simulink model "HomeAssignmentSimulinkConstants"  (R2022b)
settings: Solver=VariableStepAuto  StartTime=0.0  StopTime=6  RelTol=1e-3
settings Model: Creator=probo  LastModifiedBy=Nicher
settings DebuggingCC: UnconnectedInputMsg=warning  UnconnectedOutputMsg=warning  UnconnectedLineMsg=warning
settings ModelReferenceCC: EnableRefExpFcnMdlSchedulingChecks=on
settings RTWCC: DLArmComputeVersion=19.05

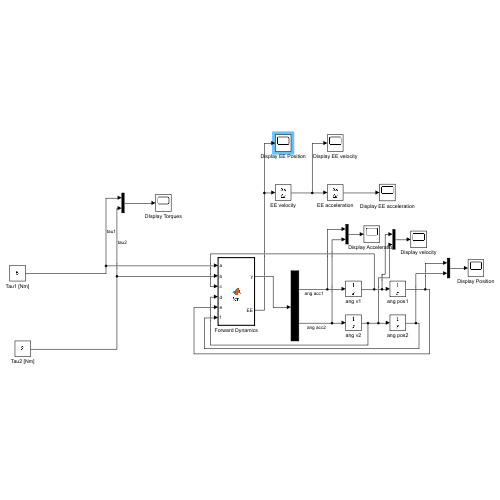
[thumbnail: Simulink's stored preview of the top-level diagram]
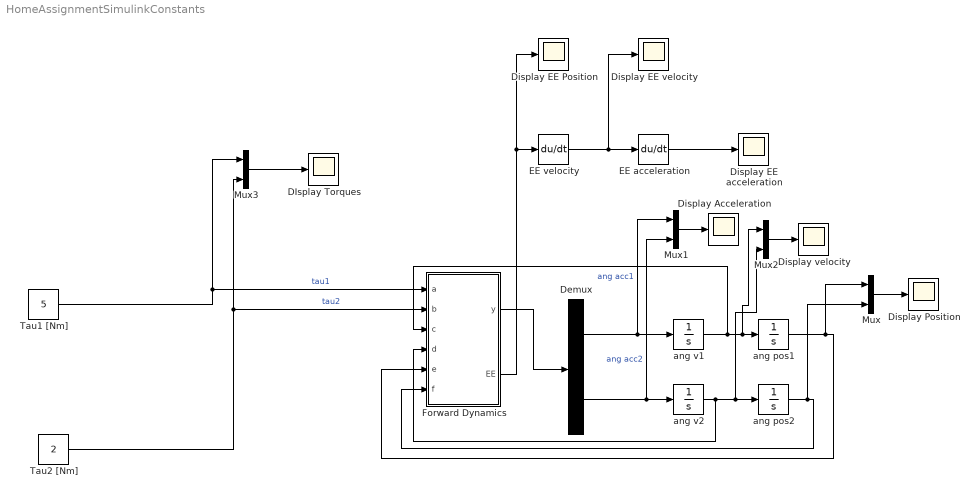
== system HomeAssignmentSimulinkConstants ==
  DIsplay Torques : Scope
  Demux : Demux  Outputs=2
  Display Acceleration : Scope
  Display EE Position : Scope
  Display EE acceleration : Scope
  Display EE velocity : Scope
  Display Position : Scope
  Display velocity : Scope
  EE acceleration : Derivative
  EE velocity : Derivative
  Forward Dynamics : MATLAB Function  TreatAsAtomicUnit=on
  Mux{,1..3} (4 alike) : Mux  Inputs=2
  Tau1 [Nm] : Constant  Value=5
  Tau2 [Nm] : Constant  Value=2
  ang pos1 : Integrator
  ang pos2 : Integrator
  ang v1 : Integrator
  ang v2 : Integrator
  wires:
  Forward Dynamics/1(y) -> Demux/1
  Demux/1 -> Mux1/1, ang v1/1  "ang acc1"
  Demux/2 -> Mux1/2, ang v2/1  "ang acc2"
  ang v1/1 -> Forward Dynamics/3(c), Mux2/1, ang pos1/1
  ang v2/1 -> Forward Dynamics/4(d), ang pos2/1, Mux2/2
  ang pos2/1 -> Mux/2, Forward Dynamics/6(f)
  ang pos1/1 -> Mux/1, Forward Dynamics/5(e)
  Mux1/1 -> Display Acceleration/1
  Mux2/1 -> Display velocity/1
  Tau2 [Nm]/1 -> Forward Dynamics/2(b), Mux3/2  "tau2"
  Tau1 [Nm]/1 -> Forward Dynamics/1(a), Mux3/1  "tau1"
  Mux3/1 -> DIsplay Torques/1
  Mux/1 -> Display Position/1
  Forward Dynamics/2(EE) -> Display EE Position/1, EE velocity/1
  EE velocity/1 -> Display EE velocity/1, EE acceleration/1
  EE acceleration/1 -> Display EE acceleration/1

== matlab function HomeAssignmentSimulinkConstants/Forward Dynamics ==
  data: a input; y output; b input; c input; d input; e input; f input; EE output
function [y, EE]= fcn(a, b, c, d, e, f)

% Torques

tau1 = a;
tau2 = b;

% Joint Velocity & Position

dtheta1 = c;
theta1 = e;

dtheta2 = d;
theta2 = f;

%Variables for link 1
l1 = 0.5;
m1 = 4.6;
I1= (1/12)*m1*l1^2;
Sc1 = [(l1/2)*cos(theta1); (l1/2)*sin(theta1); 0];
lc1 = l1/2;

Vc1 = diff(Sc1);
dVc1 = diff(Vc1);

%Variables for link 2
l2 = 0.5;
m2 = 2.3;
I2 = (1/12)*m2*l2^2;
Sc2 = [(l2/2)*cos(theta1+theta2); (l2/2)*sin(theta1+theta2); 0];
lc2 = l2/2;

Vc2 = [-l1*dtheta1*sin(theta1)-(dtheta1+dtheta2)*lc2*sin(theta1+theta2); l1*dtheta1*cos(theta1)+(dtheta1+dtheta2)*lc2*cos(theta1+theta2); 0];
dVc2 = diff(Vc2);

% Global variables

g = [
     -9.81];

S1 = [l1*cos(theta1); l1*sin(theta1)];
S2 = [l2*cos(theta1+theta2); l2*sin(theta1+theta2)];

% g Non Vector is created because normal g generates a vector inside matrix
% functions, ruining the functions that use it.
gNV = 9.81

% End effectors position

EE = (S1+S2);

% Matrix solution to forward dynamics

H11 = m1*lc1^2+I1+I2+m2*(l1^2+lc2^2+2*l1*lc2*cos(theta2));
H22 = m2*lc2^2 + I2;
H12 = m2*(lc2^2 + l1*lc2*cos(theta2))+I2;
H21 = H12;

h = m2*l1*lc2*sin(theta2);
G1 = m1*gNV*(lc1*cos(theta1)) + m2*gNV*(l1*cos(theta1) + lc2*cos(theta1 + theta2));
G2 = m2*gNV*lc2*cos(theta1 + theta2);

tau = [tau1; tau2];
M = [H11, H12; H21, H22];
V = [-h*dtheta2^2-2*h*dtheta1*dtheta2; h*dtheta1^2];
G = [G1; G2];

% Functions

%ddtheta1 = (1/I1)*(tau1-tau2-planarCross(Sc1, m1*dVc1) + planarCross(Sc1, m1*g) - planarCross(S1, m2*dVc2) + planarCross(S1, m2*g));

%ddtheta2 = (1/I2)*(tau2 - planarCross(Sc2, (m2*dVc2 - m2*g(2)))-ddtheta1);

%y = [ddtheta1;
    % ddtheta2];

ddtheta = inv(M)*(tau-(V+G))

y = ddtheta
